simulink model "SCFREYR_ADCS_toplevel"  (R2025b)
settings: Solver=FixedStepAuto  StartTime=0  StopTime=60*40  FixedStep=0.1  MaxStep=10  MinStep=1e-3  RelTol=1e-5  AbsTol=1e-5  EnableMultiTasking=on
model workspace (MAT data in the model file):
  groundstationlatitude = 45.4591667
  groundstationlongitude = -73.6383333333
  spacecraft.mass = 4.64
  spacecraft.I = [0.0114  0.0005  0.0018; 0.0005  0.0521  -1.50526e-05; 0.0018  -1.50526e-05  0.0536]
  spacecraft.orbit.a = 6786000
  spacecraft.orbit.e = 0.01
  spacecraft.orbit.inclination = 50
  spacecraft.orbit.RAAN = 95
  spacecraft.orbit.argp = 93
  spacecraft.orbit.true_anomaly = 203
  spacecraft.initial_conditions.time = 2460827.5
  spacecraft.initial_conditions.q_ff2b = [0 1 0 0]
  spacecraft.initial_conditions.w_ff2b = [0 0 0]
undefined symbols (not defined in the file or in its folder): juliandate, LP, WMM2025
libraries: simulink x14, aerolibutil x9, slpidlib x8, dspmathops x5, sharedtransform x5, simulink_extras x5, aerolibsatdyn x4, aerolibtransform2 x2, aerolibgravity2 x2, slctrl_autotuning x1, sharedutil x1, matrix_library x1
(part 1 of 2)
settings Model: Creator=The MathWorks, Inc.  LastModifiedBy=eyrns
settings SolverCC: MaxConsecutiveMinStep=10  AllowMultiTaskInputOutput=on  ConcurrentTasks=on  AutoInsertRateTranBlk=on  DecoupledContinuousIntegration=on  MinimalZcImpactIntegration=on  EnableFixedStepZeroCrossing=on  MaxZcPerStep=20.0  MaxZcBracketingIterations=30.0
settings DataIOCC: SaveFormat=StructureWithTime
settings OptimizationCC: BlockReduction=off  DefaultParameterBehavior=Inlined  BufferReuse=off  EnhancedBackFolding=on  PassReuseOutputArgsAs=Individual arguments  ZeroExternalMemoryAtStartup=off  ZeroInternalMemoryAtStartup=off  OptimizeBlockOrder=speed  DifferentSizesBufferReuse=on  EfficientTunableParamExpr=on
settings DebuggingCC: ReadBeforeWriteMsg=DisableAll  WriteAfterWriteMsg=DisableAll  WriteAfterReadMsg=DisableAll  AlgebraicLoopMsg=none  ParameterTunabilityLossMsg=error
settings ModelReferenceCC: UpdateModelReferenceTargets=IfOutOfDate  EnableRefExpFcnMdlSchedulingChecks=on
settings SFSimCC: SFSimEcho=off  MATLABDynamicMemAlloc=off
settings RTWCC: SystemTargetFile=ert.tlc  TemplateMakefile=ert_default_tmf  GPUComputeCapability=3.5  DLArmComputeVersion=19.05  Description=Embedded Coder
settings CodeAppCC: ForceParamTrailComments=on  IgnoreCustomStorageClasses=off  OperatorAnnotations=on  SimulinkDataObjDesc=on  SFDataObjDesc=on  InsertBlockDesc=on
settings ERTTargetCC: ERTCustomFileTemplate=example_file_process.tlc  TargetLangStandard=C99 (ISO)  GenerateSampleERTMain=on

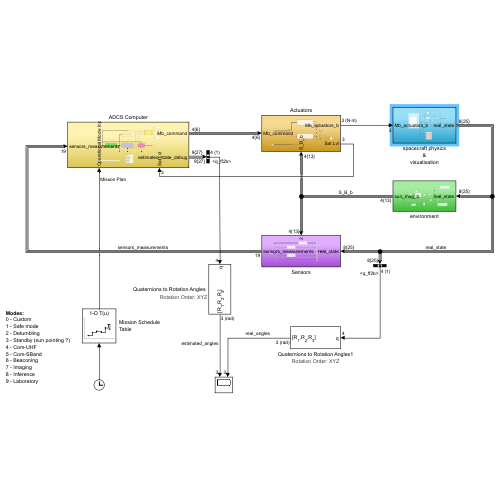
[thumbnail: Simulink's stored preview of the top-level diagram]
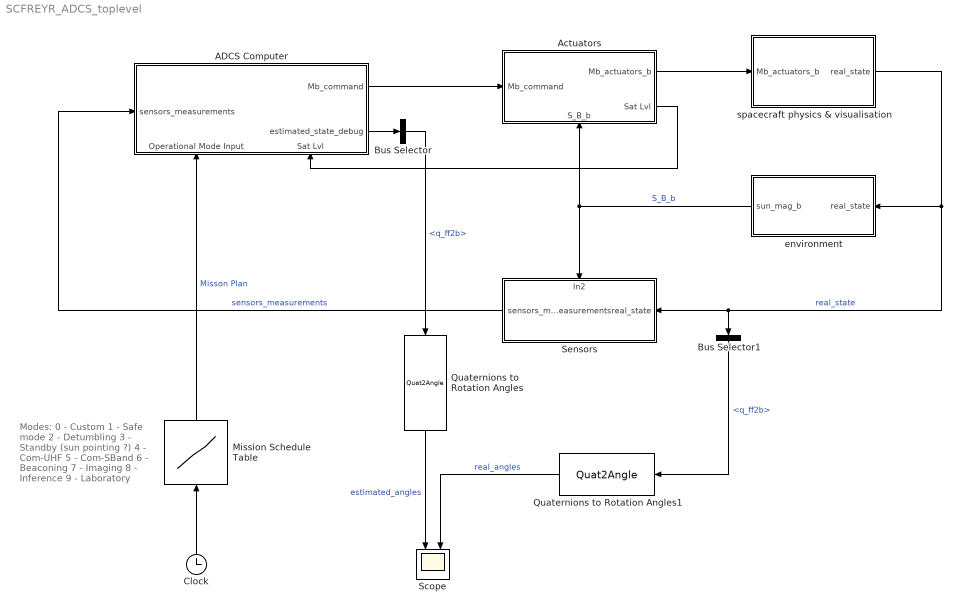
== system SCFREYR_ADCS_toplevel ==
  note: Modes:
      | 0 - Custom
      | 1 - Safe mode
      | 2 - Detumbling
      | 3 - Standby (sun pointing ?)
      | 4 - Com-UHF
      | 5 - Com-SBand
      | 6 - Beaconing
      | 7 - Imaging
      | 8 - Inference
      | 9 - Laboratory
  ADCS Computer : Subsystem
      settings: PortSchema="{\"entries\":[{\"content\":{\"sides\":[{\"content\":{\"connectorIds\":[\"In1\"]},\"type\":\"ConnectorPlacement.EquallySpacedRectSide\",\"uuid\":\"71d7f584-a1d5-4acb-9634-f2f82c6e8fe5\"},{\"content\":{\"connectorIds\":[\"Out1\",\"Out2\"],\"side\":\"RIGHT\"},\"type\":\"ConnectorPlacement.EquallySpacedRectSide\",\"uuid\":\"3e35b832-235b-44d5-94c4-e858e14eb136\"},{\"content\":{\"side\":\"TOP\"},\"type\":\"ConnectorPlacement.EquallySpacedRectSide\",\"uuid\":\"2a1d0081-a008-4252-bf57-40060fa7da55\"},{\"content\":{\"connectorIds\":[\"In2\",\"In3\"],\"side\":\"BOTTOM\"},\"type\":\"ConnectorPlacement.EquallySpacedRectSide\",\"uuid\":\"11b99e4d-157c-4c93-8086-bb24415a966e\"}]},\"type\":\"ConnectorPlacement.EquallySpacedConnector\",\"uuid\":\"b83cacd4-e2d2-442b-8aaa-4b0efa37011c\"}],\"packageUris\":[\"http://schema.mathworks.com/mf0/Connector/R2020b\"],\"version\":\"1.0\"}"
  Actuators : Subsystem
      settings: PortSchema="{\"entries\":[{\"content\":{\"sides\":[{\"content\":{\"connectorIds\":[\"In1\"]},\"type\":\"ConnectorPlacement.EquallySpacedRectSide\",\"uuid\":\"1e70e211-dd1a-4a50-a911-ed93daeec9b9\"},{\"content\":{\"connectorIds\":[\"Out1\",\"Out2\"],\"side\":\"RIGHT\"},\"type\":\"ConnectorPlacement.EquallySpacedRectSide\",\"uuid\":\"43bf107f-091b-4308-aee4-6223ab613adb\"},{\"content\":{\"side\":\"TOP\"},\"type\":\"ConnectorPlacement.EquallySpacedRectSide\",\"uuid\":\"298fd4f7-c5e8-41ca-8f54-38d83bb8d20c\"},{\"content\":{\"connectorIds\":[\"In2\"],\"side\":\"BOTTOM\"},\"type\":\"ConnectorPlacement.EquallySpacedRectSide\",\"uuid\":\"06a4a9b2-b1bf-4d6d-9e3c-15617ff96694\"}]},\"type\":\"ConnectorPlacement.EquallySpacedConnector\",\"uuid\":\"b391641d-4592-4c2b-bcae-354f2415a989\"}],\"packageUris\":[\"http://schema.mathworks.com/mf0/Connector/R2020b\"],\"version\":\"1.0\"}"
  Bus Selector : BusSelector  OutputSignals=q_ff2b
  Bus Selector1 : BusSelector  OutputSignals=q_ff2b
  Clock : Clock
  Mission Schedule Table : Lookup_n-D  NumberOfTableDimensions=1  BreakpointsForDimension1=[0 1*30 1950 2100 2400]  IndexSearchMethod=Linear search  Table=[3 3 4 3 1]  InterpMethod=Flat  ExtrapMethod=Clip  UseLastTableValue=on  InternalRulePriority=Speed  RndMeth=Simplest
  Quaternions to Rotation Angles : Quat2Angle  rotationOrder=XYZ
      settings: AttributesFormatString=Rotation Order: %<rotationOrder>
  Quaternions to Rotation Angles1 : Quat2Angle  rotationOrder=XYZ
      settings: AttributesFormatString=Rotation Order: %<rotationOrder>
  Scope : Scope  NumInputPorts=2
      settings: ActiveDisplayYMinimum=-3.9269583073309255  ActiveDisplayYMaximum=3.9266982300803996  DataLoggingVariableName=ScopeData7
  Sensors : Subsystem
      settings: PortSchema="{\"entries\":[{\"content\":{\"sides\":[{\"content\":{\"connectorIds\":[\"In1\"]},\"type\":\"ConnectorPlacement.EquallySpacedRectSide\",\"uuid\":\"1e70e211-dd1a-4a50-a911-ed93daeec9b9\"},{\"content\":{\"connectorIds\":[\"Out1\"],\"side\":\"RIGHT\"},\"type\":\"ConnectorPlacement.EquallySpacedRectSide\",\"uuid\":\"43bf107f-091b-4308-aee4-6223ab613adb\"},{\"content\":{\"connectorIds\":[\"In2\"],\"side\":\"TOP\"},\"type\":\"ConnectorPlacement.EquallySpacedRectSide\",\"uuid\":\"298fd4f7-c5e8-41ca-8f54-38d83bb8d20c\"}]},\"type\":\"ConnectorPlacement.EquallySpacedConnector\",\"uuid\":\"b391641d-4592-4c2b-bcae-354f2415a989\"}],\"packageUris\":[\"http://schema.mathworks.com/mf0/Connector/R2020b\"],\"version\":\"1.0\"}"
  environment : Subsystem
  spacecraft physics & visualisation : Subsystem
  wires:
  Actuators/1(Mb_actuators_b) -> spacecraft physics & visualisation/1(Mb_actuators_b)
  spacecraft physics & visualisation/1(real_state) -> Bus Selector1/1, Sensors/1(real_state), environment/1(real_state)  "real_state"
  Sensors/1(sensors_measurements) -> ADCS Computer/1(sensors_measurements)  "sensors_measurements"
  ADCS Computer/1(Mb_command) -> Actuators/1(Mb_command)
  environment/1(sun_mag_b) -> Actuators/2(S_B_b), Sensors/2(In2)  "S_B_b"
  ADCS Computer/2(estimated_state_debug) -> Bus Selector/1
  Bus Selector/1 -> Quaternions to Rotation Angles/1  "<q_ff2b>"
  Bus Selector1/1 -> Quaternions to Rotation Angles1/1  "<q_ff2b>"
  Quaternions to Rotation Angles1/1 -> Scope/2  "real_angles"
  Quaternions to Rotation Angles/1 -> Scope/1  "estimated_angles"
  Actuators/2(Sat Lvl) -> ADCS Computer/3(Sat Lvl)
  Mission Schedule Table/1 -> ADCS Computer/2(Operational Mode Input)  "Misson Plan"
  Clock/1 -> Mission Schedule Table/1

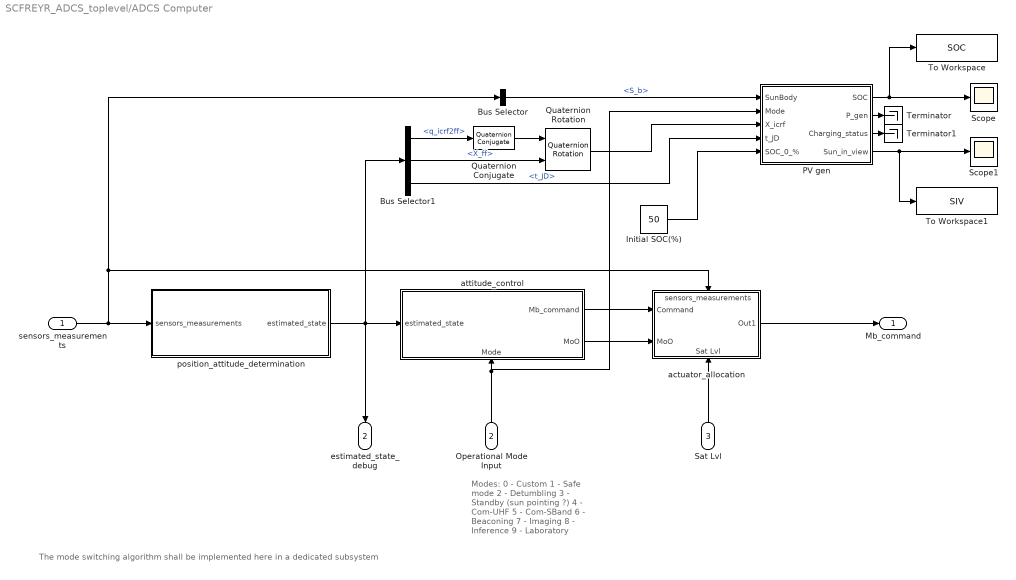
== system SCFREYR_ADCS_toplevel/ADCS Computer ==
  note: The mode switching algorithm shall be implemented here in a dedicated subsystem
  note: Modes:
      | 0 - Custom
      | 1 - Safe mode
      | 2 - Detumbling
      | 3 - Standby (sun pointing ?)
      | 4 - Com-UHF
      | 5 - Com-SBand
      | 6 - Beaconing
      | 7 - Imaging
      | 8 - Inference
      | 9 - Laboratory
  sensors_measurements : Inport
  Operational Mode Input : Inport  Port=2
  Sat Lvl : Inport  Port=3
  Bus Selector : BusSelector  OutputSignals=S_b
  Bus Selector1 : BusSelector  OutputSignals=q_icrf2ff,X_ff,t_JD
  Initial SOC(%) : Constant  Value=50
  PV gen : Subsystem
  Quaternion Conjugate : aerolibutil/Quaternion Conjugate
  Quaternion Rotation : aerolibutil/Quaternion Rotation
  Scope : Scope
      settings: ActiveDisplayYMinimum=0.483376652516037  ActiveDisplayYMaximum=0.64859278032643009  DataLoggingVariableName=ScopeData3
  Scope1 : Scope
      settings: ActiveDisplayYMinimum=0.9  ActiveDisplayYMaximum=1.1  DataLoggingVariableName=ScopeData16
  Terminator : Terminator
  Terminator1 : Terminator
  To Workspace : ToWorkspace  VariableName=SOC  SaveFormat=Timeseries  SampleTime=-1
  To Workspace1 : ToWorkspace  VariableName=SIV  SaveFormat=Timeseries  SampleTime=-1
  actuator_allocation : Subsystem
      settings: PortSchema="{\"entries\":[{\"content\":{\"sides\":[{\"content\":{\"connectorIds\":[\"In1\",\"In2\"]},\"type\":\"ConnectorPlacement.EquallySpacedRectSide\",\"uuid\":\"25120dad-b3d6-45fd-99be-bcf10d416a37\"},{\"content\":{\"connectorIds\":[\"Out1\"],\"side\":\"RIGHT\"},\"type\":\"ConnectorPlacement.EquallySpacedRectSide\",\"uuid\":\"e0cc3498-6358-4d3c-98df-bf5e9eb7cb62\"},{\"content\":{\"connectorIds\":[\"In3\"],\"side\":\"TOP\"},\"type\":\"ConnectorPlacement.EquallySpacedRectSide\",\"uuid\":\"6be13fa7-bea1-4d4d-8c61-d7ce8d494df1\"},{\"content\":{\"connectorIds\":[\"In4\"],\"side\":\"BOTTOM\"},\"type\":\"ConnectorPlacement.EquallySpacedRectSide\",\"uuid\":\"55333ee4-5cc2-40bd-af99-041699c68cf6\"}]},\"type\":\"ConnectorPlacement.EquallySpacedConnector\",\"uuid\":\"3738f58d-6af9-414b-ab0b-d496b00693c3\"}],\"packageUris\":[\"http://schema.mathworks.com/mf0/Connector/R2020b\"],\"version\":\"1.0\"}"
  attitude_control : Subsystem
      settings: PortSchema="{\"entries\":[{\"content\":{\"sides\":[{\"content\":{\"connectorIds\":[\"In1\"]},\"type\":\"ConnectorPlacement.EquallySpacedRectSide\",\"uuid\":\"7a9b0a4d-90b9-4131-b0f5-e1faac795226\"},{\"content\":{\"connectorIds\":[\"Out1\",\"Out2\"],\"side\":\"RIGHT\"},\"type\":\"ConnectorPlacement.EquallySpacedRectSide\",\"uuid\":\"a01d81c0-ef9b-4489-b3b4-96dbdcebba1c\"},{\"content\":{\"side\":\"TOP\"},\"type\":\"ConnectorPlacement.EquallySpacedRectSide\",\"uuid\":\"ab958af2-6a63-4673-8217-97c440b1739e\"},{\"content\":{\"connectorIds\":[\"In2\"],\"side\":\"BOTTOM\"},\"type\":\"ConnectorPlacement.EquallySpacedRectSide\",\"uuid\":\"0e453b5b-7699-43ce-8721-dcdf78b982dc\"}]},\"type\":\"ConnectorPlacement.EquallySpacedConnector\",\"uuid\":\"ff18fcde-34cc-4efb-867e-cd7cdf3490d9\"}],\"packageUris\":[\"http://schema.mathworks.com/mf0/Connector/R2020b\"],\"version\":\"1.0\"}"
  position_attitude_determination : Subsystem
  Mb_command : Outport
  estimated_state_debug : Outport  Port=2
  wires:
  attitude_control/1(Mb_command) -> actuator_allocation/1(Command)
  position_attitude_determination/1(estimated_state) -> Bus Selector1/1, attitude_control/1(estimated_state), estimated_state_debug/1
  sensors_measurements/1 -> actuator_allocation/3(sensors_measurements), Bus Selector/1, position_attitude_determination/1(sensors_measurements)
  actuator_allocation/1(Out1) -> Mb_command/1
  Bus Selector/1 -> PV gen/1(SunBody)  "<S_b>"
  Quaternion Conjugate/1 -> Quaternion Rotation/1
  Bus Selector1/1 -> Quaternion Conjugate/1  "<q_icrf2ff>"
  Bus Selector1/2 -> Quaternion Rotation/2  "<X_ff>"
  Quaternion Rotation/1 -> PV gen/3(X_icrf)
  PV gen/1(SOC) -> To Workspace/1, Scope/1
  Bus Selector1/3 -> PV gen/4(t_JD)  "<t_JD>"
  Initial SOC(%)/1 -> PV gen/5(SOC_0_%)
  PV gen/2(P_gen) -> Terminator/1
  PV gen/3(Charging_status) -> Terminator1/1
  PV gen/4(Sun_in_view) -> To Workspace1/1, Scope1/1
  Operational Mode Input/1 -> PV gen/2(Mode), attitude_control/2(Mode)
  Sat Lvl/1 -> actuator_allocation/4(Sat Lvl)
  attitude_control/2(MoO) -> actuator_allocation/2(MoO)

== system SCFREYR_ADCS_toplevel/Actuators ==
  Mb_command : Inport
  S_B_b : Inport  Port=2
  Bus Selector : BusSelector  OutputSignals=RW,MT
  Bus Selector1 : BusSelector  OutputSignals=B_b
  Magnetorquers : Subsystem
      settings: PortSchema="{\"entries\":[{\"content\":{\"sides\":[{\"content\":{\"connectorIds\":[\"In1\"]},\"type\":\"ConnectorPlacement.EquallySpacedRectSide\",\"uuid\":\"1e70e211-dd1a-4a50-a911-ed93daeec9b9\"},{\"content\":{\"connectorIds\":[\"Out1\"],\"side\":\"RIGHT\"},\"type\":\"ConnectorPlacement.EquallySpacedRectSide\",\"uuid\":\"43bf107f-091b-4308-aee4-6223ab613adb\"},{\"content\":{\"side\":\"TOP\"},\"type\":\"ConnectorPlacement.EquallySpacedRectSide\",\"uuid\":\"298fd4f7-c5e8-41ca-8f54-38d83bb8d20c\"},{\"content\":{\"connectorIds\":[\"In2\"],\"side\":\"BOTTOM\"},\"type\":\"ConnectorPlacement.EquallySpacedRectSide\",\"uuid\":\"6bb05069-049a-46db-950a-a10972af5c08\"}]},\"type\":\"ConnectorPlacement.EquallySpacedConnector\",\"uuid\":\"b391641d-4592-4c2b-bcae-354f2415a989\"}],\"packageUris\":[\"http://schema.mathworks.com/mf0/Connector/R2020b\"],\"version\":\"1.0\"}"
  Mux : Mux  Inputs=2
  Reaction wheels : Subsystem
  Sum : Sum  Inputs=+|+
  Torques : Scope  NumInputPorts=2
      settings: ActiveDisplayYMinimum=-0.00029476333864894506  ActiveDisplayYMaximum=0.00029342808107133751  DataLoggingVariableName=ScopeData21
  Mb_actuators_b : Outport
  Sat Lvl : Outport  Port=2
  wires:
  Bus Selector/1 -> Reaction wheels/1(RW_b)  "<RW>"
  Bus Selector/2 -> Magnetorquers/1(M_MT_b_command)  "<MT>"
  Sum/1 -> Torques/1, Mb_actuators_b/1  "Total"
  Reaction wheels/1(M_RW_b) -> Mux/1, Sum/1  "M_RW_b"
  Magnetorquers/1(M_MT_b) -> Mux/2, Sum/2  "M_MT_b"
  S_B_b/1 -> Bus Selector1/1
  Bus Selector1/1 -> Magnetorquers/2(B_b)  "<B_b>"
  Mb_command/1 -> Bus Selector/1
  Reaction wheels/2(Sat Lvl) -> Sat Lvl/1
  Mux/1 -> Torques/2

== system SCFREYR_ADCS_toplevel/Sensors ==
  real_state : Inport
  In2 : Inport  Port=2
  Bus Creator : BusCreator  Inputs=5
  Bus Selector : BusSelector  OutputSignals=S_b,q_icrf2ff,B_b,V_ff
  Gyro : Subsystem
  Magnetometer : Subsystem
  Sunsensor : Subsystem
  sensors_measurements : Outport
  wires:
  real_state/1 -> Gyro/1(In1)
  Bus Creator/1 -> sensors_measurements/1
  Sunsensor/1(S_b_sensor) -> Bus Creator/2  "S_b"
  Magnetometer/1(B_b_sensor) -> Bus Creator/4  "B_b"
  Gyro/1(Out1) -> Bus Creator/1  "Gyro Data"
  In2/1 -> Bus Selector/1
  Bus Selector/3 -> Magnetometer/1(B_b)  "<B_b>"
  Bus Selector/1 -> Sunsensor/1(S_b)  "<S_b>"
  Bus Selector/2 -> Bus Creator/3  "<q_icrf2ff>"
  Bus Selector/4 -> Bus Creator/5  "<V_ff>"

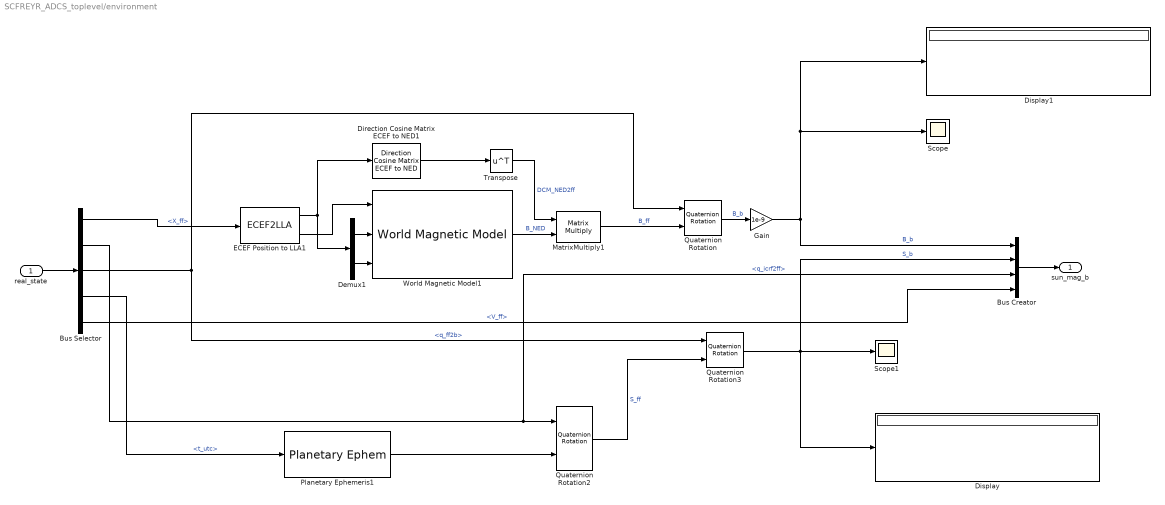
== system SCFREYR_ADCS_toplevel/environment ==
  real_state : Inport
  Bus Creator : BusCreator  Inputs=4
  Bus Selector : BusSelector  OutputSignals=X_ff,q_icrf2ff,q_ff2b,t_utc,V_ff
  Demux1 : Demux  Outputs=2
  Direction Cosine Matrix ECEF to NED1 : aerolibtransform2/Direction Cosine Matrix ECEF to NED
  Display : Display
  Display1 : Display
  ECEF Position to LLA1 : ECEF2LLA
  Gain : Gain  Gain=1e-9
  MatrixMultiply1 : Product  Multiplication=Matrix(*)
  Planetary Ephemeris1 : PlanetaryEphem  ephemerisModel=DE421  target=Sun  outputVelocity=off
  Quaternion Rotation : aerolibutil/Quaternion Rotation
  Quaternion Rotation2 : aerolibutil/Quaternion Rotation
  Quaternion Rotation3 : aerolibutil/Quaternion Rotation
  Scope : Scope
      settings: ActiveDisplayYMinimum=-47080.06600486581  ActiveDisplayYMaximum=48448.675094254395
  Scope1 : Scope
      settings: ActiveDisplayYMinimum=-6.6630089033459878  ActiveDisplayYMaximum=7.9356738417232382
  Transpose : Math  Operator=transpose
  World Magnetic Model1 : aerolibgravity2/World Magnetic Model  model=WMM2025 (2025-2030)  customFile='WMM2025.COF'  units=Metric (MKS)  time_in=off  month=January  day=1  year=2026  action=Error  h_out=off  dec_out=off  inc_out=off  ti_out=off
  sun_mag_b : Outport
  wires:
  Bus Selector/1 -> ECEF Position to LLA1/1  "<X_ff>"
  Bus Selector/4 -> Planetary Ephemeris1/1  "<t_utc>"
  real_state/1 -> Bus Selector/1
  Bus Creator/1 -> sun_mag_b/1
  Quaternion Rotation/1 -> Gain/1  "B_b"
  Bus Selector/3 -> Quaternion Rotation3/1, Quaternion Rotation/1  "<q_ff2b>"
  Planetary Ephemeris1/1 -> Quaternion Rotation2/2
  Quaternion Rotation2/1 -> Quaternion Rotation3/2  "S_ff"
  Bus Selector/2 -> Bus Creator/3, Quaternion Rotation2/1  "<q_icrf2ff>"
  Quaternion Rotation3/1 -> Display/1, Bus Creator/2, Scope1/1  "S_b"
  Direction Cosine Matrix ECEF to NED1/1 -> Transpose/1
  Demux1/1 -> World Magnetic Model1/2
  MatrixMultiply1/1 -> Quaternion Rotation/2  "B_ff"
  Transpose/1 -> MatrixMultiply1/1  "DCM_NED2ff"
  Demux1/2 -> World Magnetic Model1/3
  ECEF Position to LLA1/1 -> Demux1/1, Direction Cosine Matrix ECEF to NED1/1
  World Magnetic Model1/1 -> MatrixMultiply1/2  "B_NED"
  ECEF Position to LLA1/2 -> World Magnetic Model1/1
  Gain/1 -> Scope/1, Display1/1, Bus Creator/1  "B_b"
  Bus Selector/5 -> Bus Creator/4  "<V_ff>"

== system SCFREYR_ADCS_toplevel/spacecraft physics & visualisation ==
  note: Spacecraft Plant
  note: Observation
  Mb_actuators_b : Inport
  Bus Creator : BusCreator  Inputs=8
  Degrees to Radians : simulink_extras/Transformations/Degrees to Radians
  Degrees to Radians1 : simulink_extras/Transformations/Degrees to Radians
  Quaternion Multiplication : aerolibutil/Quaternion Multiplication
  Quaternions to Rotation Angles : Quat2Angle  rotationOrder=XYZ
      settings: AttributesFormatString=Rotation Order: %<rotationOrder>
  Satellite Scenario Playback : Subsystem  StopFcn=|  mask{openViewer=on, stateFrame=ECEF (Fixed-frame), useVelocity=on, useAttitude=on, attitudeFrame=ECEF (Fixed-frame), satName=SC-FREYR, showTriad=on, show3dModel=on, showFOV=on, fovHalfAngle=30, scenarioStep=60}
      | exSatScenBlk = gcb;
      | exSatScenMdl = bdroot(exSatScenBlk);
      | 
      | % If workspace blocks are stored in single output variable, need to access from there
      | if get_param(exSatScenMdl, "ReturnWorkspaceOutputs") == "on"
      |     exSatScenOutVar = get_param(exSatScenMdl, "ReturnWorkspaceOutputsName");
      |     if exist(exSatScenOutVar)
      |         exSatScenTimeData = eval(exSatScenOutVar).exSatScenTimeData;
      |         exSatScenPositionData = eval(exSatScenOutVar).exSatScenPositionData;
      |         exSatScenVelocityData = eval(exSatScenOutVar).exSatScenVelocityData;
      |         exSatScenAttitudeData = eval(exSatScenOutVar).exSatScenAttitudeData;
      |     end
      | end
      | 
      | % If variables exist, create scenario (variables are not created if called with sim command)
      | if exist("exSatScenTimeData") && exist("exSatScenPositionData") && exist("exSatScenVelocityData") && exist("exSatScenAttitudeData") 
      |     % Create satellite scenario from variables accessed above or directly from workspace
      |     exSatScenario = Aero.spacecraft.analysis.createSatelliteScenarioFromSim(exSatScenBlk, ...
      |         exSatScenTimeData, exSatScenPositionData, exSatScenVelocityData, exSatScenAttitudeData);
      | end
      | 
      | clear exSatScenBlk exSatScenMdl exSatScenOutVar exSatScenTimeData exSatScenPositionData exSatScenVelocityData exSatScenAttitudeData
      mask prompts: openViewer "Enable Satellite Scenario Viewer playback animation"; stateFrame "State coordinate frame:"; useVelocity "Add velocity port"; useAttitude "Add attitude port"; attitudeFrame "Attitude coordinate frame (Frame to Body):"; satName "Satellite or constellation label:"; showTriad "Show coordinate axis triad (Body frame)"; show3dModel "Show 3D satellite model"; showFOV "Add sensor field-of-view (FOV)"; fovHalfAngle "FOV half angle (deg):"; scenarioStep "Satellite scenario sample time (s):"
      mask init:
      | ports = Aero.spacecraft.analysis.satelliteScenarioPlaybackMaskCallback(gcb, "init");
      settings: AttributesFormatString=Open viewer: %<openViewer>
      mask Callback openViewer: Aero.spacecraft.analysis.satelliteScenarioPlaybackMaskCallback(gcb, "viewer");
      mask TypeOptions stateFrame: Inertial (ICRF) | ECEF (Fixed-frame) | Geographic
      mask Callback useAttitude: Aero.spacecraft.analysis.satelliteScenarioPlaybackMaskCallback(gcb, "attitude");
      mask TypeOptions attitudeFrame: Inertial (ICRF) | ECEF (Fixed-frame) | NED
      mask Callback showFOV: Aero.spacecraft.analysis.satelliteScenarioPlaybackMaskCallback(gcb, "fov");
      mask DialogControl DescGroupVar Prompt: Satellite Scenario Viewer Playback Animation
      mask DialogControl DescTextVar Prompt: <html><p>Create a satellite scenario object and launch the Satellite Scenario Viewer using the trajectories provided as inputs to the block.</p><p>If playback animation is enabled, the block opens Satellite Scenario Viewer after the model simulation has stopped. The viewer will not launch if the model is run using the <tt>sim</tt> command.</p> <p>To add additional satellites, ground stations, or platforms to the scenario and perform mission analysis, including line-of-sight access and eclipse analysis, use the base workspace variable <tt>exSatScenario</tt>.</p></html>
      mask DialogControl Container3 Prompt: Parameters
      mask DialogControl Container4 Prompt: Trajectory
      mask DialogControl ParameterGroupVar Prompt: Playback
      mask DialogControl SatelliteScenarioPlaybackTag Prompt: SatelliteScenarioPlaybackTag
      mask Display:
      | port_label(ports(1).type,ports(1).port,ports(1).txt,'texmode','on');
      | port_label(ports(2).type,ports(2).port,ports(2).txt,'texmode','on');
      | port_label(ports(3).type,ports(3).port,ports(3).txt,'texmode','on');
      | port_label(ports(4).type,ports(4).port,ports(4).txt,'texmode','on');
  Scope : Scope  NumInputPorts=3
      settings: ActiveDisplayYMinimum=-3.9269456980970325  ActiveDisplayYMaximum=3.9269473746794858  DataLoggingVariableName=ScopeData24
  Spacecraft Dynamics : SpacecraftDynamics  forcesIn=off  accelFrame=Fixed-frame  outportFrame=Fixed-frame  outputAccel=on  startDate=spacecraft.initial_conditions.time  mass=spacecraft.mass  inertia=spacecraft.I  semiMajorAxis=spacecraft.orbit.a  eccentricity=spacecraft.orbit.e  inclination=spacecraft.orbit.inclination  raan=spacecraft.orbit.RAAN  argPeriapsis=spacecraft.orbit.argp  trueAnomaly=spacecraft.orbit.true_anomaly  attitudeFrame=Fixed-frame  attitude=spacecraft.initial_conditions.q_ff2b  attitudeRate=spacecraft.initial_conditions.w_ff2b  outputAngAccel=on  outputTransform=on  dragArea=0.03  ephemerisModel=DE421  useThirdBodyGravity=on  moonThirdBodyGravityModel=Spherical harmonics  moonThirdBodySH=LP-165P  moonThirdBodySHDegree=120
  Terminator : Terminator
  real_state : Outport
  wires:
  Spacecraft Dynamics/8 -> Satellite Scenario Playback/1(timeInput), Bus Creator/7  "t_utc"
  Spacecraft Dynamics/2 -> Satellite Scenario Playback/3(velocityInput), Bus Creator/2  "V_ff"
  Spacecraft Dynamics/4 -> Satellite Scenario Playback/4(attitudeInput), Quaternion Multiplication/1, Bus Creator/3  "q_ff2b"
  Bus Creator/1 -> real_state/1
  Spacecraft Dynamics/7 -> Quaternion Multiplication/2, Bus Creator/4  "q_icrf2ff"
  Spacecraft Dynamics/1 -> Satellite Scenario Playback/2(positionInput), Bus Creator/1  "X_ff"
  Spacecraft Dynamics/5 -> Bus Creator/6, Degrees to Radians/1  "w_ff2b"
  Quaternion Multiplication/1 -> Quaternions to Rotation Angles/1, Bus Creator/5  "q_icrf2b"
  Spacecraft Dynamics/3 -> Terminator/1
  Degrees to Radians/1 -> Scope/2
  Degrees to Radians1/1 -> Scope/3
  Quaternions to Rotation Angles/1 -> Scope/1
  Spacecraft Dynamics/6 -> Bus Creator/8, Degrees to Radians1/1  "alpha_icrf2b"
  Mb_actuators_b/1 -> Spacecraft Dynamics/1

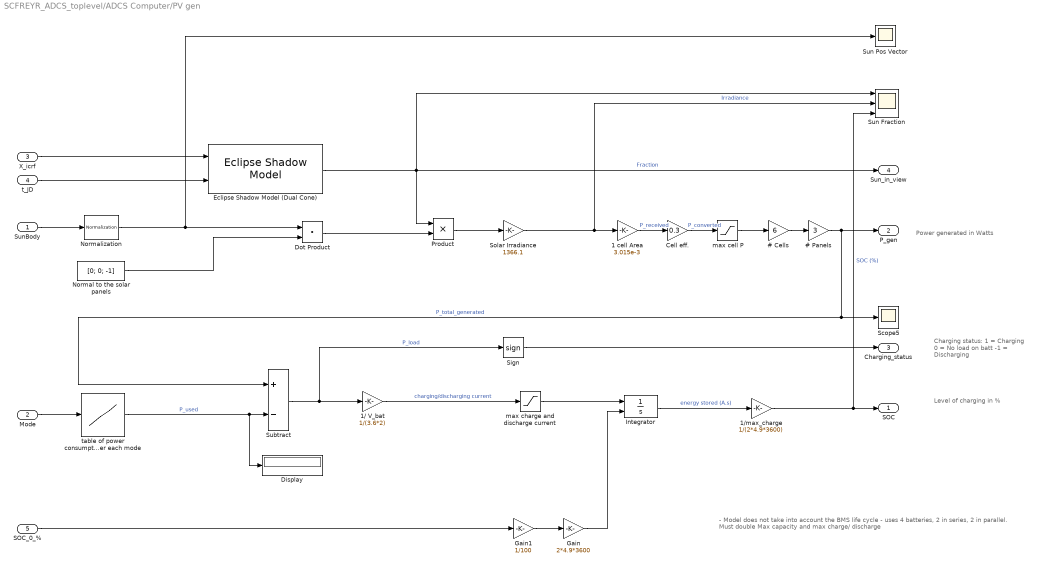
== system SCFREYR_ADCS_toplevel/ADCS Computer/PV gen ==
  note: Level of charging in %
  note: Power generated in Watts
  note: Charging status:
      | 1 = Charging
      | 0 = No load on batt
      | -1 = Discharging
  note: - Model does not take into account the BMS life cycle
      | - uses 4 batteries, 2 in series, 2 in parallel. Must double Max capacity and max charge/
      | discharge
  SunBody : Inport
  Mode : Inport  Port=2
  X_icrf : Inport  Port=3
  t_JD : Inport  Port=4
  SOC_0_% : Inport  Port=5
  # Cells : Gain  Gain=6
  # Panels : Gain  Gain=3
  1 cell Area : Gain  Gain=3.015e-3
  1/ V_bat : Gain  Gain=1/(3.6*2)
  1/max_charge : Gain  Gain=1/(2*4.9*3600)
  Cell eff. : Gain  Gain=0.3
  Display : Display
  Dot Product : DotProduct  OutDataTypeStr=Inherit: Inherit via internal rule
  Eclipse Shadow Model (Dual Cone) : EclipseShadowModel  timeSource=Port (Julian date)  startDate=juliandate(2025, 1, 1)  useEphemerisDateRange=off  ephemerisStartDate=juliandate(2025, 1, 1)
  Gain : Gain  Gain=2*4.9*3600
  Gain1 : Gain  Gain=1/100
  Integrator : Integrator  InitialConditionSource=external  InitialCondition=2*4.9*3600  LimitOutput=on  UpperSaturationLimit=2*4.9*3600  LowerSaturationLimit=0
  Normal to the solar panels : Constant  Value=[0; 0; -1]
  Normalization : dspmathops/Normalization  NormType=2-norm  Bias=1e-10  NormOver=Each row  Dimension=1  roundingMode=Floor  overflowMode=off  accumDataTypeStr=Inherit: Same as product output  accumLastDataTypeStr=Inherit: Same as product output  outputDataTypeStr=Inherit: Same as product output  outputMin=[]  outputMax=[]  outputLastDataTypeStr=Inherit: Same as product output
  Product : Product
  Scope5 : Scope
      settings: ActiveDisplayYMinimum=-2.7674999999999996  ActiveDisplayYMaximum=24.9075  DataLoggingVariableName=ScopeData6
  Sign : Signum
  Solar Irradiance : Gain  Gain=1366.1
  Subtract : Sum  Inputs=+-
  Sun Fraction : Scope  NumInputPorts=3
      settings: ActiveDisplayYMinimum=219.573674026196  ActiveDisplayYMaximum=545.69684821697467
  Sun Pos Vector : Scope
      settings: ActiveDisplayYMinimum=-1.2478722130486144  ActiveDisplayYMaximum=1.245094841150906  DataLoggingVariableName=ScopeData3
  max cell P : Saturate  UpperLimit=1.23  LowerLimit=0
  max charge and discharge current : Saturate  UpperLimit=(2*2.45)  LowerLimit=-(2*4.9)
  table of power consumption per each mode : Lookup_n-D  NumberOfTableDimensions=1  BreakpointsForDimension1=[0, 1, 2, 3, 4, 5, 6, 7, 8, 9]  Table=[0, 2.2, 4.93, 5.32, 8.97, 12.44, 8.66, 10.93, 11.79, 6.86]  InternalRulePriority=Speed  RndMeth=Simplest
  SOC : Outport
  P_gen : Outport  Port=2
  Charging_status : Outport  Port=3
  Sun_in_view : Outport  Port=4
  wires:
  table of power consumption per each mode/1 -> Display/1, Subtract/2  "P_used"
  # Panels/1 -> Subtract/1, Scope5/1, P_gen/1  "P_total_generated"
  Subtract/1 -> Sign/1, 1/ V_bat/1  "P_load"
  Integrator/1 -> 1/max_charge/1  "energy stored (A.s)"
  1/max_charge/1 -> Sun Fraction/3, SOC/1  "SOC (%)"
  SunBody/1 -> Normalization/1
  max cell P/1 -> # Cells/1
  Cell eff./1 -> max cell P/1  "P_converted"
  X_icrf/1 -> Eclipse Shadow Model (Dual Cone)/1
  Eclipse Shadow Model (Dual Cone)/1 -> Product/1, Sun_in_view/1, Sun Fraction/1  "Fraction"
  # Cells/1 -> # Panels/1
  1 cell Area/1 -> Cell eff./1  "P_received"
  Solar Irradiance/1 -> Sun Fraction/2, 1 cell Area/1  "Irradiance"
  Mode/1 -> table of power consumption per each mode/1
  max charge and discharge current/1 -> Integrator/1
  1/ V_bat/1 -> max charge and discharge current/1  "charging/discharging current"
  Sign/1 -> Charging_status/1
  t_JD/1 -> Eclipse Shadow Model (Dual Cone)/2
  Gain1/1 -> Gain/1
  Gain/1 -> Integrator/2
  SOC_0_%/1 -> Gain1/1
  Product/1 -> Solar Irradiance/1
  Normalization/1 -> Dot Product/1, Sun Pos Vector/1
  Normal to the solar panels/1 -> Dot Product/2
  Dot Product/1 -> Product/2

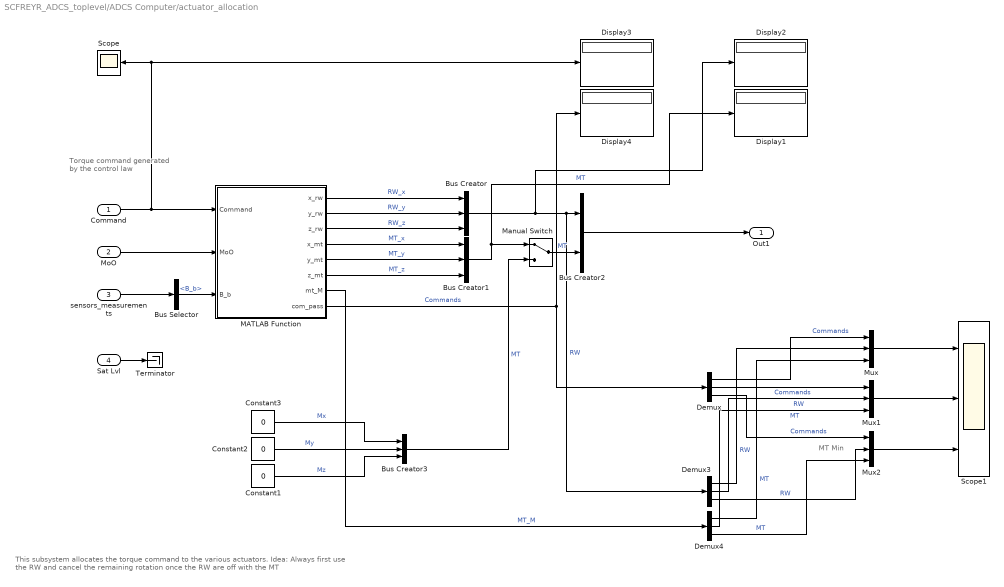
== system SCFREYR_ADCS_toplevel/ADCS Computer/actuator_allocation ==
  note: MT Min
  note: This subsystem allocates the torque command to the various actuators.
      | Idea: Always first use the RW and cancel the remaining rotation once the RW are off with the MT
  note: Torque command generated by the control law
  Command : Inport
  MoO : Inport  Port=2
  sensors_measurements : Inport  Port=3
  Sat Lvl : Inport  Port=4
  Bus Creator : BusCreator  Inputs=3
  Bus Creator1 : BusCreator  Inputs=3
  Bus Creator2 : BusCreator  Inputs=2
  Bus Creator3 : BusCreator  Inputs=3
  Bus Selector : BusSelector  OutputSignals=B_b
  Constant1 : Constant  Value=0
  Constant2 : Constant  Value=0
  Constant3 : Constant  Value=0
  Demux : Demux  Outputs=3
  Demux3 : Demux  Outputs=3
  Demux4 : Demux  Outputs=3
  Display{1..4} (4 alike) : Display
  MATLAB Function : MATLAB Function  TreatAsAtomicUnit=on
  Manual Switch : ManualSwitch
  Mux : Mux  Inputs=3
  Mux1 : Mux  Inputs=3
  Mux2 : Mux  Inputs=3
  Scope : Scope
      settings: ActiveDisplayYMinimum=-0.009553279032749171  ActiveDisplayYMaximum=0.0059795112947425367  DataLoggingVariableName=ScopeData9
  Scope1 : Scope  NumInputPorts=3
      settings: ActiveDisplayString=3  ActiveDisplayYMinimum=-67.0961577709568  ActiveDisplayYMaximum=10.555618707265149  DataLoggingVariableName=ScopeData25
  Terminator : Terminator
  Out1 : Outport
  wires:
  Manual Switch/1 -> Bus Creator2/2  "MT"
  Bus Creator3/1 -> Manual Switch/2  "MT"
  Constant1/1 -> Bus Creator3/3  "Mz"
  Constant2/1 -> Bus Creator3/2  "My"
  Constant3/1 -> Bus Creator3/1  "Mx"
  Bus Creator2/1 -> Out1/1
  Command/1 -> Display3/1, Scope/1, MATLAB Function/1(Command)
  Sat Lvl/1 -> Terminator/1
  sensors_measurements/1 -> Bus Selector/1
  MATLAB Function/1(x_rw) -> Bus Creator/1  "RW_x"
  MATLAB Function/2(y_rw) -> Bus Creator/2  "RW_y"
  MATLAB Function/4(x_mt) -> Bus Creator1/1  "MT_x"
  MATLAB Function/5(y_mt) -> Bus Creator1/2  "MT_y"
  MATLAB Function/6(z_mt) -> Bus Creator1/3  "MT_z"
  Bus Creator1/1 -> Display1/1, Manual Switch/1  "MT"
  MATLAB Function/3(z_rw) -> Bus Creator/3  "RW_z"
  Bus Creator/1 -> Demux3/1, Bus Creator2/1, Display2/1  "RW"
  MATLAB Function/8(com_pass) -> Demux/1, Display4/1  "Commands"
  Demux/1 -> Mux/1  "Commands"
  Demux/2 -> Mux1/1  "Commands"
  Demux/3 -> Mux2/1  "Commands"
  Demux3/1 -> Mux/2  "RW"
  Demux3/2 -> Mux1/2  "RW"
  Demux3/3 -> Mux2/2  "RW"
  Demux4/1 -> Mux/3  "MT"
  Demux4/2 -> Mux1/3  "MT"
  Demux4/3 -> Mux2/3  "MT"
  Mux/1 -> Scope1/1
  Mux1/1 -> Scope1/2
  Mux2/1 -> Scope1/3
  MoO/1 -> MATLAB Function/2(MoO)
  MATLAB Function/7(mt_M) -> Demux4/1  "MT_M"
  Bus Selector/1 -> MATLAB Function/3(B_b)  "<B_b>"

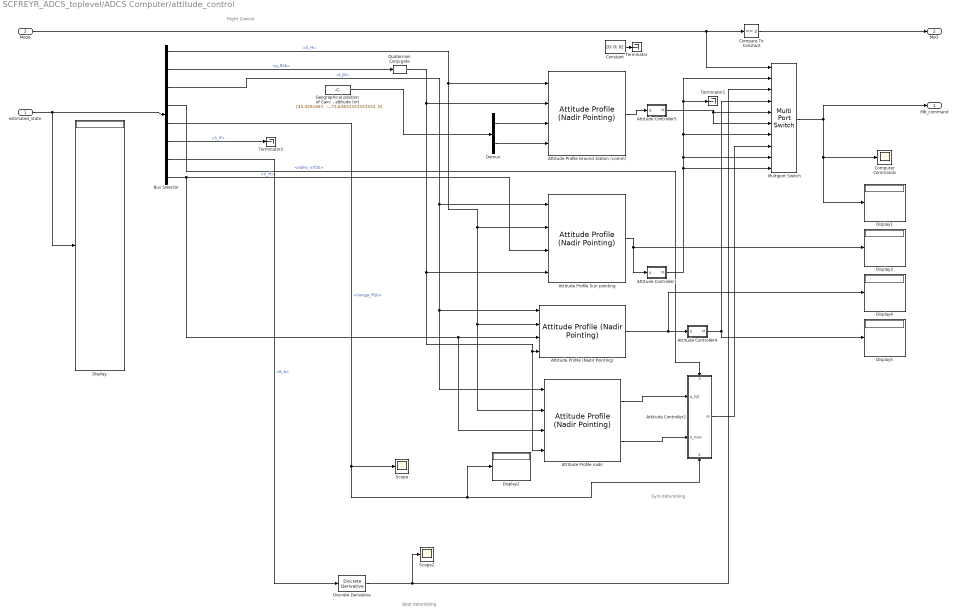
== system SCFREYR_ADCS_toplevel/ADCS Computer/attitude_control ==
  note: Gyro detumbling
  note: Bdot detumbling
  note: Flight Control
  estimated_state : Inport
  Mode : Inport  Port=2
  Attitude Controller1 : Subsystem
  Attitude Controller2 : Subsystem
      settings: PortSchema="{\"entries\":[{\"content\":{\"sides\":[{\"content\":{\"connectorIds\":[\"In1\",\"In2\"]},\"type\":\"ConnectorPlacement.EquallySpacedRectSide\",\"uuid\":\"0ec87e19-81a9-48a5-b369-4e5979653f17\"},{\"content\":{\"connectorIds\":[\"Out1\"],\"side\":\"RIGHT\"},\"type\":\"ConnectorPlacement.EquallySpacedRectSide\",\"uuid\":\"07bba412-4f91-4e53-8458-d82370bbd40d\"},{\"content\":{\"connectorIds\":[\"In3\"],\"side\":\"TOP\"},\"type\":\"ConnectorPlacement.EquallySpacedRectSide\",\"uuid\":\"47129328-3243-497a-93d5-70fbb6bc0035\"},{\"content\":{\"connectorIds\":[\"In4\"],\"side\":\"BOTTOM\"},\"type\":\"ConnectorPlacement.EquallySpacedRectSide\",\"uuid\":\"b45e8311-6252-42fb-8b0f-653ef2d8563f\"}]},\"type\":\"ConnectorPlacement.EquallySpacedConnector\",\"uuid\":\"916ee354-dd78-4f6a-83d4-fc0930c110e9\"}],\"packageUris\":[\"http://schema.mathworks.com/mf0/Connector/R2020b\"],\"version\":\"1.0\"}"
  Attitude Controller4 : Subsystem
  Attitude Controller5 : Subsystem
  Attitude Profile (Nadir Pointing) : aerolibsatdyn/Attitude Profile (Nadir Pointing)  outputError=on  outputFinalAttitude=off  portFrame=Fixed-frame  pointingMode=Point at nadir  celestialTarget=Sun  tunablePointing=off  primaryAlignmentSrc=Dialog  primaryAlignment=[0 1 0]  secondaryAlignmentSrc=Dialog  secondaryAlignment=[0 0 1]  constraintFrame=LVLH  primaryConstraintSrc=Dialog  primaryConstraint=[1 0 0]  secondaryConstraintSrc=Dialog  secondaryConstraint=[0 1 0]
  Attitude Profile Ground station (comm) : aerolibsatdyn/Attitude Profile (Nadir Pointing)  outputError=on  outputFinalAttitude=off  portFrame=Fixed-frame  pointingMode=Point at LatLonAlt  celestialTarget=Sun  tunablePointing=off  primaryAlignmentSrc=Dialog  primaryAlignment=[0 1 0]  secondaryAlignmentSrc=Dialog  secondaryAlignment=[1 0 0]  constraintFrame=Fixed-frame  primaryConstraintSrc=Dialog  primaryConstraint=[1 0 0]  secondaryConstraintSrc=Dialog  secondaryConstraint=[0 1 0]
  Attitude Profile Sun pointing : aerolibsatdyn/Attitude Profile (Nadir Pointing)  outputError=on  outputFinalAttitude=off  portFrame=Fixed-frame  pointingMode=Point at celestial body  celestialTarget=Sun  tunablePointing=off  primaryAlignmentSrc=Dialog  primaryAlignment=[0 -1 0]  secondaryAlignmentSrc=Dialog  secondaryAlignment="[0  0 1]"  constraintFrame=LVLH  primaryConstraintSrc=Dialog  primaryConstraint=[0 1 0]  secondaryConstraintSrc=Dialog  secondaryConstraint=[0 1 0]
  Attitude Profile nadir : aerolibsatdyn/Attitude Profile (Nadir Pointing)  outputError=on  outputFinalAttitude=on  portFrame=Fixed-frame  pointingMode=Point at nadir  celestialTarget=Sun  tunablePointing=off  primaryAlignmentSrc=Dialog  primaryAlignment=[0 -1 0]  secondaryAlignmentSrc=Dialog  secondaryAlignment=[0 0 1]  constraintFrame=LVLH  primaryConstraintSrc=Dialog  primaryConstraint=[1 0 0]  secondaryConstraintSrc=Dialog  secondaryConstraint=[0 1 0]
  Bus Selector : BusSelector  OutputSignals=X_ff,q_ff2b,t_JD,Gyro Data.alpha_icrf2b,Gyro Data.omega_ff2b,S_ff,B_b,V_ff
  Compare To Constant : simulink/Logic and Bit Operations/Compare To Constant  relop===  const=2  OutDataTypeStr=boolean
  Computer Commands : Scope
      settings: ActiveDisplayYMinimum=-0.009553279032749171  ActiveDisplayYMaximum=0.0059795112947425367  DataLoggingVariableName=ScopeData14
  Constant : Constant  Value=[0; 0; 0]
  Demux : Demux  Outputs=[2 1]
  Discrete Derivative : simulink/Discrete/Discrete Derivative  gainval=1.0  ICPrevScaledInput=0.0  OutMin=[]  OutMax=[]  OutDataType=fixdt(1, 16)  OutScaling=2^-10  DoSatur=off
  Display{,1..5} (6 alike) : Display
      Display3 settings: Decimation=3
      Display4 settings: Decimation=3
      Display5 settings: Decimation=3
  "Geographical position of Campus Loyola Latitude (deg), Longitude (deg), altitude (m)" : Constant  Value=[45.4591667, -73.63833333333334, 0]
  Multiport Switch : MultiPortSwitch  Inputs=9  SaturateOnIntegerOverflow=off  InputSameDT=off
  Quaternion Conjugate : aerolibutil/Quaternion Conjugate
  Scope : Scope
      settings: ActiveDisplayYMinimum=-3.7524837013413928  ActiveDisplayYMaximum=1.4887264309797046  DataLoggingVariableName=ScopeData13
  Scope2 : Scope
      settings: ActiveDisplayYMinimum=-9.1599816403475832E-7  ActiveDisplayYMaximum=2.0382352836057713E-6  DataLoggingVariableName=ScopeData18
  Terminator : Terminator
  Terminator1 : Terminator
  Terminator2 : Terminator
  Mb_command : Outport
  MoO : Outport  Port=2
  wires:
  Quaternion Conjugate/1 -> Attitude Profile nadir/4, Attitude Profile (Nadir Pointing)/4, Attitude Profile Sun pointing/4, Attitude Profile Ground station (comm)/2
  Attitude Profile Ground station (comm)/1 -> Attitude Controller5/1(q)
  Demux/2 -> Attitude Profile Ground station (comm)/4
  Attitude Profile nadir/1 -> Attitude Controller2/1(q_tgt)
  Demux/1 -> Attitude Profile Ground station (comm)/3
  "Geographical position of Campus Loyola Latitude (deg), Longitude (deg), altitude (m)"/1 -> Demux/1
  Attitude Profile Sun pointing/1 -> Attitude Controller1/1(q), Display3/1
  Mode/1 -> Multiport Switch/1, Compare To Constant/1
  Bus Selector/5 -> Display2/1, Attitude Controller2/4(<omega_ff2b>), Scope/1  "<omega_ff2b>"
  Bus Selector/2 -> Quaternion Conjugate/1  "<q_ff2b>"
  Bus Selector/1 -> Attitude Profile nadir/2, Attitude Profile (Nadir Pointing)/2, Attitude Profile Sun pointing/2, Attitude Profile Ground station (comm)/1  "<X_ff>"
  Multiport Switch/1 -> Display1/1, Computer Commands/1, Mb_command/1
  Attitude Controller5/1(M) -> Multiport Switch/6, Multiport Switch/5
  Attitude Controller1/1(M) -> Multiport Switch/7, Terminator1/1, Multiport Switch/2, Multiport Switch/9, Multiport Switch/10
  Bus Selector/7 -> Discrete Derivative/1  "<B_b>"
  Discrete Derivative/1 -> Multiport Switch/3, Scope2/1
  Constant/1 -> Terminator/1
  Attitude Controller2/1(M) -> Multiport Switch/8
  Attitude Profile nadir/2 -> Attitude Controller2/2(q_new)
  Bus Selector/4 -> Attitude Controller2/3(<alpha_icrf2b>)  "<alpha_icrf2b>"
  estimated_state/1 -> Display/1, Bus Selector/1
  Attitude Profile (Nadir Pointing)/1 -> Display4/1, Attitude Controller4/1(q)
  Attitude Controller4/1(M) -> Multiport Switch/4, Display5/1
  Bus Selector/8 -> Attitude Profile (Nadir Pointing)/3, Attitude Profile nadir/3, Attitude Profile Sun pointing/3  "<V_ff>"
  Bus Selector/3 -> Attitude Profile nadir/1, Attitude Profile (Nadir Pointing)/1, Attitude Profile Sun pointing/1  "<t_JD>"
  Bus Selector/6 -> Terminator2/1  "<S_ff>"
  Compare To Constant/1 -> MoO/1

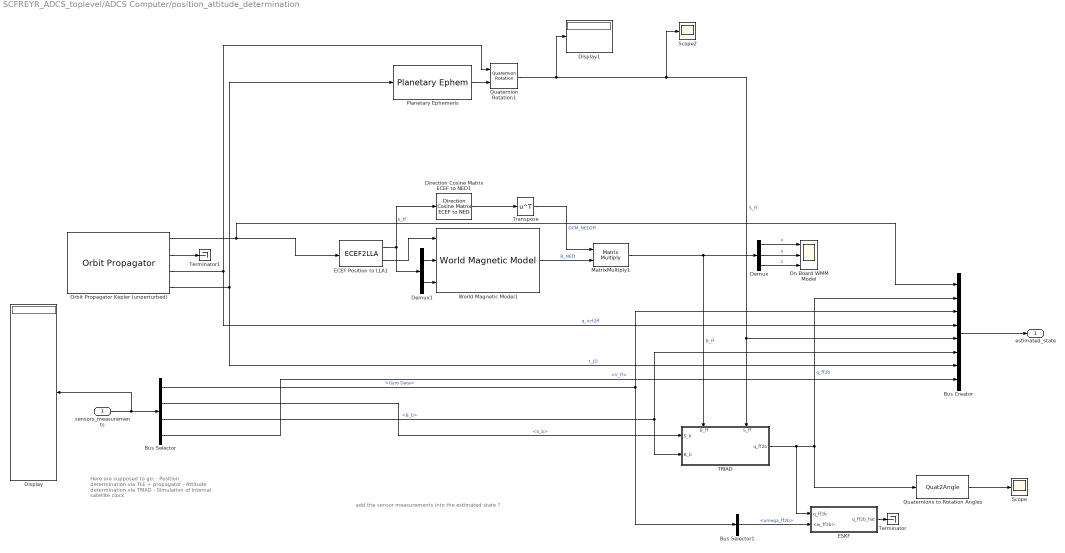
== system SCFREYR_ADCS_toplevel/ADCS Computer/position_attitude_determination ==
  note: Here are supposed to go:
      | - Position determination via TLE + propagator
      | - Attitude determination via TRIAD
      | - Simulation of internal satellite clock
  note: add the sensor measurements into the estimated state ?
  sensors_measurements : Inport
  Bus Creator : BusCreator  Inputs=8
  Bus Selector : BusSelector  OutputSignals=Gyro Data,S_b,B_b,V_ff
  Bus Selector1 : BusSelector  OutputSignals=omega_ff2b
  Demux : Demux  Outputs=3
  Demux1 : Demux  Outputs=2
  Direction Cosine Matrix ECEF to NED1 : aerolibtransform2/Direction Cosine Matrix ECEF to NED
  Display : Display
  Display1 : Display
  ECEF Position to LLA1 : ECEF2LLA
  ESKF : Subsystem
  MatrixMultiply1 : Product  Multiplication=Matrix(*)
  On Board WMM Model : Scope  NumInputPorts=3
      settings: ActiveDisplayYMinimum=-53544.234529387868  ActiveDisplayYMaximum=50242.730513721755  DataLoggingVariableName=ScopeData4
  Orbit Propagator Kepler (unperturbed) : OrbitPropagator  propagator=Numerical (high precision)  outportFrame=Fixed-frame  startDate=spacecraft.initial_conditions.time  mass=spacecraft.mass  semiMajorAxis=spacecraft.orbit.a  eccentricity=spacecraft.orbit.e  inclination=spacecraft.orbit.inclination  raan=spacecraft.orbit.RAAN  argPeriapsis=spacecraft.orbit.argp  trueAnomaly=spacecraft.orbit.true_anomaly  inertialPosition=[3649700.0 3308200.0 -4676600.0]  inertialVelocity=[-2750.8 6666.4 2573.4]  fixedPosition=[-4142689.0 -2676864.7 -4669861.6]  fixedVelocity=[1452.7 -6720.7 2568.1]  customR=3396200  customMu=4.305e13  customJ2=1.0826269e-03  customOmega=4.06125949e-3  shDegree=10  outputTransform=on  useDrag=on  dragArea=0.03  useSRP=on  srpArea=0.5
  Planetary Ephemeris : PlanetaryEphem  ephemerisModel=DE421  target=Sun  outputVelocity=off
  Quaternion Rotation1 : aerolibutil/Quaternion Rotation
  Quaternions to Rotation Angles : Quat2Angle  rotationOrder=XYZ
      settings: AttributesFormatString=Rotation Order: %<rotationOrder>
  Scope : Scope
      settings: ActiveDisplayYMinimum=-3.9263388642364703  ActiveDisplayYMaximum=5.07457557405816  DataLoggingVariableName=ScopeData2
  Scope2 : Scope
      settings: ActiveDisplayYMinimum=-2.0387726478323829E+8  ActiveDisplayYMaximum=7.0333981760995939E+7  DataLoggingVariableName=ScopeData6
  TRIAD : Subsystem
      settings: PortSchema="{\"entries\":[{\"content\":{\"sides\":[{\"content\":{\"connectorIds\":[\"In1\",\"In2\"]},\"type\":\"ConnectorPlacement.EquallySpacedRectSide\",\"uuid\":\"934d396e-f242-4144-8e49-7dca4c529b1e\"},{\"content\":{\"connectorIds\":[\"Out1\"],\"side\":\"RIGHT\"},\"type\":\"ConnectorPlacement.EquallySpacedRectSide\",\"uuid\":\"d5049cd6-8da5-467a-a595-0659620b3453\"},{\"content\":{\"connectorIds\":[\"In3\",\"In4\"],\"side\":\"TOP\"},\"type\":\"ConnectorPlacement.EquallySpacedRectSide\",\"uuid\":\"566a2326-4576-4247-b03e-f5181e2b65c9\"}]},\"type\":\"ConnectorPlacement.EquallySpacedConnector\",\"uuid\":\"3190049e-3c9f-4103-9960-cf9fc3914e67\"}],\"packageUris\":[\"http://schema.mathworks.com/mf0/Connector/R2020b\"],\"version\":\"1.0\"}"
  Terminator : Terminator
  Terminator1 : Terminator
  Transpose : Math  Operator=transpose
  World Magnetic Model1 : aerolibgravity2/World Magnetic Model  model=WMM2025 (2025-2030)  customFile='WMM2025.COF'  units=Metric (MKS)  time_in=off  month=January  day=1  year=2026  action=Error  h_out=off  dec_out=off  inc_out=off  ti_out=off
  estimated_state : Outport
  wires:
  Bus Creator/1 -> estimated_state/1
  Orbit Propagator Kepler (unperturbed)/1 -> ECEF Position to LLA1/1, Bus Creator/1  "X_ff"
  Orbit Propagator Kepler (unperturbed)/4 -> Planetary Ephemeris/1, Bus Creator/7  "t_JD"
  Quaternion Rotation1/1 -> Display1/1, TRIAD/4(S_ff), Bus Creator/5, Scope2/1  "S_ff"
  sensors_measurements/1 -> Display/1, Bus Selector/1
  Bus Selector/1 -> Bus Selector1/1, Bus Creator/3  "<Gyro Data>"
  Bus Selector/3 -> TRIAD/2(B_b), Bus Creator/6  "<B_b>"
  Bus Selector/2 -> TRIAD/1(S_b)  "<S_b>"
  TRIAD/1(q_ff2b) -> ESKF/1(q_ff2b), Quaternions to Rotation Angles/1, Bus Creator/2  "q_ff2b"
  Quaternions to Rotation Angles/1 -> Scope/1
  ESKF/1(q_ff2b_hat) -> Terminator/1
  Orbit Propagator Kepler (unperturbed)/2 -> Terminator1/1
  Direction Cosine Matrix ECEF to NED1/1 -> Transpose/1
  Demux1/1 -> World Magnetic Model1/2
  Transpose/1 -> MatrixMultiply1/1  "DCM_NED2ff"
  Demux1/2 -> World Magnetic Model1/3
  ECEF Position to LLA1/1 -> Demux1/1, Direction Cosine Matrix ECEF to NED1/1
  World Magnetic Model1/1 -> MatrixMultiply1/2  "B_NED"
  ECEF Position to LLA1/2 -> World Magnetic Model1/1
  MatrixMultiply1/1 -> Demux/1, TRIAD/3(B_ff)  "B_ff"
  Planetary Ephemeris/1 -> Quaternion Rotation1/2
  Orbit Propagator Kepler (unperturbed)/3 -> Bus Creator/4, Quaternion Rotation1/1  "q_icrf2ff"
  Demux/1 -> On Board WMM Model/1  "x"
  Demux/2 -> On Board WMM Model/2  "y"
  Demux/3 -> On Board WMM Model/3  "z"
  Bus Selector1/1 -> ESKF/2(<w_ff2b>)  "<omega_ff2b>"
  Bus Selector/4 -> Bus Creator/8  "<V_ff>"

== system SCFREYR_ADCS_toplevel/Actuators/Magnetorquers ==
  M_MT_b_command : Inport
  B_b : Inport  Port=2
  Cross Product : matrix_library/Cross Product
  M_MT_b : Outport
  wires:
  M_MT_b_command/1 -> Cross Product/2
  B_b/1 -> Cross Product/1
  Cross Product/1 -> M_MT_b/1  "M"

== system SCFREYR_ADCS_toplevel/Actuators/Reaction wheels ==
  RW_b : Inport
  Display : Display
  Reaction wheels : Subsystem
  Scope1 : Scope
      settings: ActiveDisplayYMinimum=-0.00029162125950114994  ActiveDisplayYMaximum=0.00031019074600742295  DataLoggingVariableName=ScopeData5
  M_RW_b : Outport
  Sat Lvl : Outport  Port=2
  wires:
  RW_b/1 -> Reaction wheels/1(M_desired)
  Reaction wheels/2(M_generated) -> M_RW_b/1, Scope1/1
  Reaction wheels/1(issat) -> Display/1
  Reaction wheels/3(Sat Lvl) -> Sat Lvl/1

== system SCFREYR_ADCS_toplevel/Sensors/Gyro ==
  In1 : Inport
  Bus Creator : BusCreator  Inputs=2
  Bus Selector : BusSelector  OutputSignals=w_ff2b,alpha_icrf2b
  Constant : Constant  Value=[0; 0; 0]
  Display : Display  Commented=on
  Manual Switch : ManualSwitch
  Random Number : RandomNumber  Variance=75e-3 * 75e-3  SampleTime=0
  Sum : Sum  Inputs=|++
  Out1 : Outport
  wires:
  In1/1 -> Bus Selector/1
  Bus Selector/1 -> Sum/1  "<w_ff2b>"
  Sum/1 -> Bus Creator/1, Display/1  "omega_ff2b"
  Random Number/1 -> Manual Switch/2
  Constant/1 -> Manual Switch/1
  Manual Switch/1 -> Sum/2
  Bus Selector/2 -> Bus Creator/2  "<alpha_icrf2b>"
  Bus Creator/1 -> Out1/1

== system SCFREYR_ADCS_toplevel/Sensors/Magnetometer ==
  B_b : Inport
  Constant : Constant  Value=[0; 0; 0]
  Manual Switch : ManualSwitch
  Random Number : RandomNumber  Variance=20*20  SampleTime=0
  Scope : Scope
      settings: ActiveDisplayYMinimum=-110.5218379536206  ActiveDisplayYMaximum=140.35483561949053  DataLoggingVariableName=ScopeData15
  Scope1 : Scope
      settings: ActiveDisplayYMinimum=-3.5167376363783974E-5  ActiveDisplayYMaximum=4.9021953923482364E-5  DataLoggingVariableName=ScopeData17
  Sum : Sum  Inputs=++|
  B_b_sensor : Outport
  wires:
  B_b/1 -> Sum/2
  Sum/1 -> Scope1/1, B_b_sensor/1
  Random Number/1 -> Scope/1, Manual Switch/2
  Manual Switch/1 -> Sum/1
  Constant/1 -> Manual Switch/1

== system SCFREYR_ADCS_toplevel/Sensors/Sunsensor ==
  S_b : Inport
  Display : Display
  Scope : Scope
      settings: ActiveDisplayYMinimum=-1.8900558135338327E+8  ActiveDisplayYMaximum=1.8416392195937455E+8  DataLoggingVariableName=ScopeData12
  S_b_sensor : Outport
  wires:
  S_b/1 -> S_b_sensor/1, Scope/1, Display/1

== system SCFREYR_ADCS_toplevel/spacecraft physics & visualisation/Satellite Scenario Playback ==
  timeInput : Inport  PortDimensions=1
  positionInput : Inport  Port=2  Unit=m
  velocityInput : Inport  Port=3  Unit=m/s
  attitudeInput : Inport  Port=4
  AttitudeDataOut : ToWorkspace  VariableName=exSatScenAttitudeData  SampleTime=-1
  Check att dimensions : Subsystem  mask{N=4, AssertionFailFcn=error("Attitude input must be be a vector with 4 elements or a 2-D array of size [m x 4].")}
      mask prompts: N "State dimension (N):"; AssertionFailFcn "Simulink:blkprm_prompts:AssertionCallback"
      mask TypeOptions AssertionFailFcn: Assertion/AssertionFailFcn | Second check/Assertion/AssertionFailFcn
      mask DialogControl DescGroupVar Prompt: Assert expected dimensions
      mask DialogControl DescTextVar Prompt: Assert that input signal is size N or size M x N where M is the number of satellites. N is 3 for position and velocity, and 4 for attitude (quaternions).
      mask DialogControl AssertionFailFcn Prompt: Simulation callback when assertion fails:
  Check pos dimensions : Subsystem  mask{N=3, AssertionFailFcn=error("Position input must be be a vector with 3 elements or a 2-D array of size [m x 3].")}
      mask prompts: N "State dimension (N):"; AssertionFailFcn "Simulink:blkprm_prompts:AssertionCallback"
      mask TypeOptions AssertionFailFcn: Assertion/AssertionFailFcn | Second check/Assertion/AssertionFailFcn
      mask DialogControl DescGroupVar Prompt: Assert expected dimensions
      mask DialogControl DescTextVar Prompt: Assert that input signal is size N or size M x N where M is the number of satellites. N is 3 for position and velocity, and 4 for attitude (quaternions).
      mask DialogControl AssertionFailFcn Prompt: Simulation callback when assertion fails:
  Check vel dimensions : Subsystem  mask{N=3, AssertionFailFcn=error("Velocity input must be be a vector with 3 elements or a 2-D array of size [m x 3].")}
      mask prompts: N "State dimension (N):"; AssertionFailFcn "Simulink:blkprm_prompts:AssertionCallback"
      mask TypeOptions AssertionFailFcn: Assertion/AssertionFailFcn | Second check/Assertion/AssertionFailFcn
      mask DialogControl DescGroupVar Prompt: Assert expected dimensions
      mask DialogControl DescTextVar Prompt: Assert that input signal is size N or size M x N where M is the number of satellites. N is 3 for position and velocity, and 4 for attitude (quaternions).
      mask DialogControl AssertionFailFcn Prompt: Simulation callback when assertion fails:
  PositionDataOut : ToWorkspace  VariableName=exSatScenPositionData  SampleTime=-1
  TimeDataOut : ToWorkspace  VariableName=exSatScenTimeData  SampleTime=-1
  VelocityDataOut : ToWorkspace  VariableName=exSatScenVelocityData  SampleTime=-1
  wires:
  positionInput/1 -> PositionDataOut/1, Check pos dimensions/1(input)
  velocityInput/1 -> Check vel dimensions/1(input), VelocityDataOut/1
  attitudeInput/1 -> Check att dimensions/1(input), AttitudeDataOut/1
  timeInput/1 -> TimeDataOut/1
